simulink model "closeloopteori"  (R2015b)
settings: Solver=VariableStepAuto  StartTime=0.0  StopTime=10.0  RelTol=1e-3
settings Model: Creator=wafiq  LastModifiedBy=wafiq

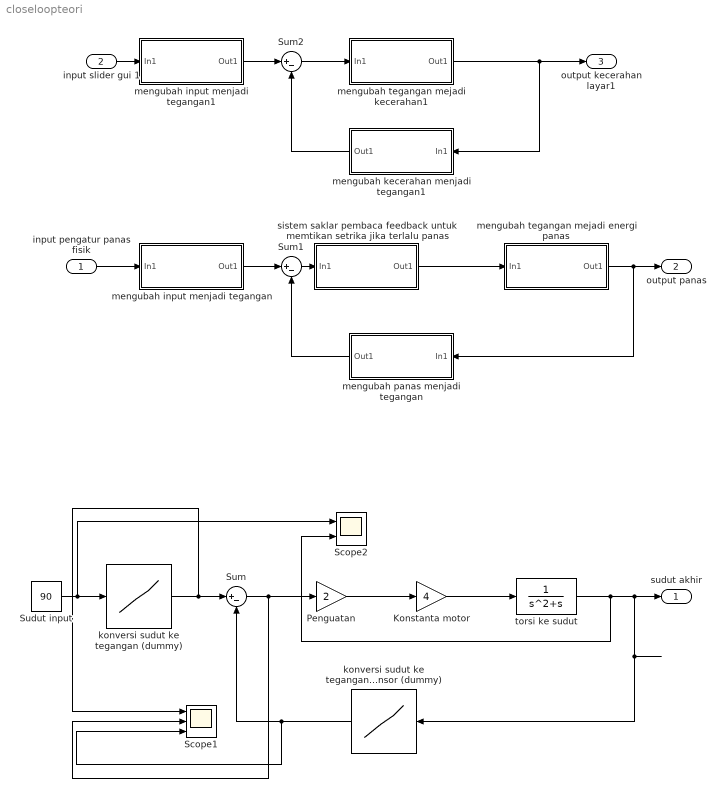
== system closeloopteori ==
  input pengatur panas fisik : Inport
  input slider gui 1 : Inport  Port=2
  Konstanta motor : Gain  Gain=4
  Penguatan : Gain  Gain=2
  Scope1 : Scope  NumInputPorts=3
  Scope2 : Scope  NumInputPorts=2
  "Sudut input " : Constant  Value=90
  Sum : Sum  Inputs=|+-
  Sum1 : Sum  Inputs=|+-
  Sum2 : Sum  Inputs=|+-
  konversi sudut ke tegangan (dummy) : Lookup_n-D  NumberOfTableDimensions=1  BreakpointsForDimension1=[36,72,108,180,216,252,288,324,360,400,480]  Table=[5,5.5,6,6.6,7,7.5,8,8.5,9,12,15]  InternalRulePriority=Speed  RndMeth=Simplest  InputSameDT=on
  konversi sudut ke tegangan pada sensor (dummy) : Lookup_n-D  NumberOfTableDimensions=1  BreakpointsForDimension1=[36,72,108,180,216,252,288,324,360,400,480]  Table=[5,5.5,6,6.6,7,7.5,8,8.5,9,12,15]  InternalRulePriority=Speed  RndMeth=Simplest  InputSameDT=on
  mengubah input menjadi tegangan : Subsystem
  mengubah input menjadi tegangan1 : Subsystem
  mengubah kecerahan menjadi tegangan1 : Subsystem
  mengubah panas menjadi tegangan : Subsystem
  mengubah tegangan mejadi energi panas : Subsystem
  mengubah tegangan mejadi kecerahan1 : Subsystem
  sistem saklar pembaca feedback untuk memtikan setrika jika terlalu panas : Subsystem
  torsi ke sudut : TransferFcn  Denominator=[1 1 0]
  sudut akhir : Outport
  output panas : Outport  Port=2
  output kecerahan layar1 : Outport  Port=3
  wires:
  konversi sudut ke tegangan (dummy)/1 -> Scope1/1, Sum/1
  "Sudut input "/1 -> Scope2/1, konversi sudut ke tegangan (dummy)/1
  torsi ke sudut/1 -> Scope2/2, konversi sudut ke tegangan pada sensor (dummy)/1, sudut akhir/1
  konversi sudut ke tegangan pada sensor (dummy)/1 -> Scope1/3, Sum/2
  Penguatan/1 -> Konstanta motor/1
  Konstanta motor/1 -> torsi ke sudut/1
  mengubah panas menjadi tegangan/1(Out1) -> Sum1/2
  mengubah input menjadi tegangan/1(Out1) -> Sum1/1
  input pengatur panas fisik/1 -> mengubah input menjadi tegangan/1(In1)
  mengubah tegangan mejadi energi panas/1(Out1) -> mengubah panas menjadi tegangan/1(In1), output panas/1
  mengubah kecerahan menjadi tegangan1/1(Out1) -> Sum2/2
  Sum2/1 -> mengubah tegangan mejadi kecerahan1/1(In1)
  mengubah input menjadi tegangan1/1(Out1) -> Sum2/1
  input slider gui 1/1 -> mengubah input menjadi tegangan1/1(In1)
  mengubah tegangan mejadi kecerahan1/1(Out1) -> mengubah kecerahan menjadi tegangan1/1(In1), output kecerahan layar1/1
  Sum1/1 -> sistem saklar pembaca feedback untuk memtikan setrika jika terlalu panas/1(In1)
  sistem saklar pembaca feedback untuk memtikan setrika jika terlalu panas/1(Out1) -> mengubah tegangan mejadi energi panas/1(In1)
  Sum/1 -> Scope1/2, Penguatan/1

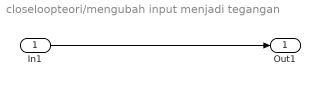
== system closeloopteori/mengubah input menjadi tegangan ==
  In1 : Inport
  Out1 : Outport
  wires:
  In1/1 -> Out1/1

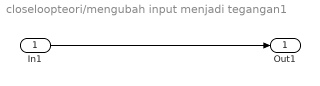
== system closeloopteori/mengubah input menjadi tegangan1 ==
  In1 : Inport
  Out1 : Outport
  wires:
  In1/1 -> Out1/1

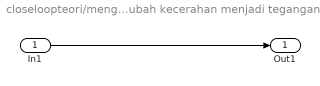
== system closeloopteori/mengubah kecerahan menjadi tegangan1 ==
  In1 : Inport
  Out1 : Outport
  wires:
  In1/1 -> Out1/1

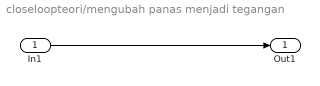
== system closeloopteori/mengubah panas menjadi tegangan ==
  In1 : Inport
  Out1 : Outport
  wires:
  In1/1 -> Out1/1

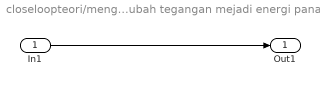
== system closeloopteori/mengubah tegangan mejadi energi panas ==
  In1 : Inport
  Out1 : Outport
  wires:
  In1/1 -> Out1/1

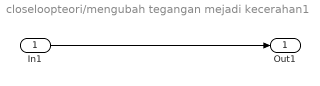
== system closeloopteori/mengubah tegangan mejadi kecerahan1 ==
  In1 : Inport
  Out1 : Outport
  wires:
  In1/1 -> Out1/1

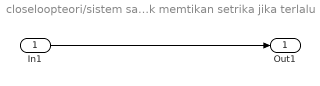
== system closeloopteori/sistem saklar pembaca feedback untuk memtikan setrika jika terlalu panas ==
  In1 : Inport
  Out1 : Outport
  wires:
  In1/1 -> Out1/1
